simulink model "pcm_multimedia"  (R2018a)
settings: Solver=VariableStepAuto  StartTime=0.0  StopTime=10.0  RelTol=1e-3
libraries: dsparch4 x2, commutil2 x2, dspquant2 x2, dspvision x1, dspsigops x1
settings Model: Creator=hp  LastModifiedBy=hp

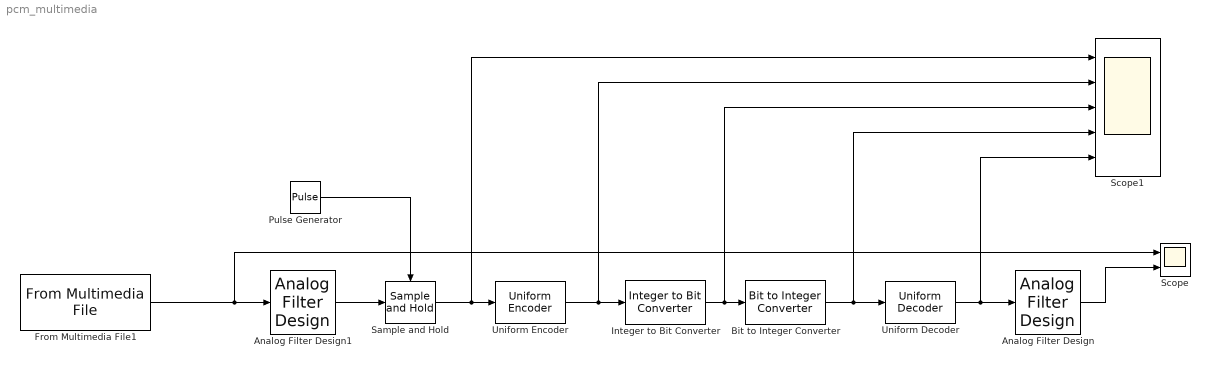
== system pcm_multimedia ==
  Analog Filter Design : dsparch4/Analog Filter Design  method=Butterworth  filttype=Bandpass  N=8  Wlo=2*pi*300  Whi=2*pi*3400  Rp=2  Rs=40
  Analog Filter Design1 : dsparch4/Analog Filter Design  method=Butterworth  filttype=Bandpass  N=8  Wlo=2*pi*300  Whi=2*pi*3400  Rp=2  Rs=40
  Bit to Integer Converter : commutil2/Bit to Integer Converter  nbits=8  bitOrder=MSB first  signedOutputValues=Unsigned  outDtype=Inherit via internal rule  outDtypeSigned=Inherit via internal rule
  From Multimedia File1 : dspvision/From Multimedia File  inputFilename=C:\Program Files\MATLAB\R2018a\toolbox\dsp\dsp\dspafxf_8000.wav  loop=on  numPlays=inf  outputStreams=Audio only  videoDataType=single  audioDataType=double  inheritSampleTime=on  userDefinedSampleTime=1/30  noAudioOutput=off  isIntensityVideo=off  fourcc=RGB  colorVideoFormat=Separate color signals  outputEOF=off  dataOrg=Column-major  audioFrameSize=1  computeAudioFrameSize=off  outSamplingMode=Sample based
      settings: SourceProductBaseCode=VP
  Integer to Bit Converter : commutil2/Integer to Bit Converter  nbits=8  signedInputValues=Unsigned  bitOrder=MSB first  outDtype=Inherit via internal rule
  Pulse Generator : DiscretePulseGenerator  PulseType=Time based  Period=1/8000  PulseWidth=50
  Sample and Hold : dspsigops/Sample and Hold  trig=Rising edge  initCond=0  latchinput=off
  Scope : Scope  NumInputPorts=2
  Scope1 : Scope  NumInputPorts=5
  Uniform Decoder : dspquant2/Uniform Decoder  peak=1  bits=8  overflowMode=Saturate  otype=Double
      settings: SourceProductName=DSP System Toolbox  SourceProductBaseCode=DS
  Uniform Encoder : dspquant2/Uniform Encoder  peak=1  bits=8  otype=Unsigned integer
      settings: SourceProductName=DSP System Toolbox
  wires:
  Uniform Decoder/1 -> Scope1/5, Analog Filter Design/1
  Bit to Integer Converter/1 -> Scope1/4, Uniform Decoder/1
  Integer to Bit Converter/1 -> Scope1/3, Bit to Integer Converter/1
  Analog Filter Design/1 -> Scope/2
  Uniform Encoder/1 -> Scope1/2, Integer to Bit Converter/1
  Sample and Hold/1 -> Scope1/1, Uniform Encoder/1
  Pulse Generator/1 -> Sample and Hold/Trigger
  Analog Filter Design1/1 -> Sample and Hold/1
  From Multimedia File1/1 -> Scope/1, Analog Filter Design1/1
